simulink model "LineFollowing3kush"  (R2023a)
settings: Solver=FixedStepDiscrete  StartTime=0.0  StopTime=500  FixedStep=0.01  RelTol=1e-3
undefined symbols (not defined in the file or in its folder): InputPWM, WheelSpeed
libraries: arduinolib x10, commrandsrc3 x1, arduinosensorlib x1
settings Model: SimulationMode=external  ExtModeTrigDuration=2  Creator=Boitumelo  LastModifiedBy=ankus
settings SolverCC: AutoInsertRateTranBlk=on
settings OptimizationCC: EnhancedBackFolding=on  PassReuseOutputArgsAs=Individual arguments  ZeroExternalMemoryAtStartup=off  ZeroInternalMemoryAtStartup=off  MaxStackSize=64  OptimizeBlockOrder=speed  DifferentSizesBufferReuse=on  OptimizationCustomize=off  EfficientTunableParamExpr=on
settings DebuggingCC: ParameterTunabilityLossMsg=error  UnconnectedInputMsg=warning  UnconnectedOutputMsg=warning  UnconnectedLineMsg=warning
settings HardwareCC: ProdBitPerPointer=32  ProdBitPerSizeT=32  ProdBitPerPtrDiffT=32  ProdLargestAtomicInteger=Long  ProdLargestAtomicFloat=Double  ProdWordSize=32  ProdHWDeviceType=ARM Compatible->ARM Cortex
settings SFSimCC: MATLABDynamicMemAlloc=off
settings RTWCC: Description=Embedded Coder  SystemTargetFile=ert.tlc  HardwareBoard=Arduino Nano 33 IoT  TemplateMakefile=ert_default_tmf  GenerateReport=on  RTWVerbose=off  RTWUseSimCustomCode=on  Toolchain=Arduino ARM  BuildConfiguration=Faster Runs  DLArmComputeVersion=19.05
settings CodeAppCC: ForceParamTrailComments=on  IgnoreCustomStorageClasses=off  MaxIdLength=32  OperatorAnnotations=on  SimulinkDataObjDesc=on  SFDataObjDesc=on  InsertBlockDesc=on
settings ERTTargetCC: SupportContinuousTime=on  SupportVariableSizeSignals=on  ExtModeTransport=3  ExtModeStaticAlloc=on  ExtModeAutomaticAllocSize=off  ExtModeStaticAllocSize=8192  ExtModeMexFile=ext_xcp  ExtModeIntrfLevel=Level2 - Open

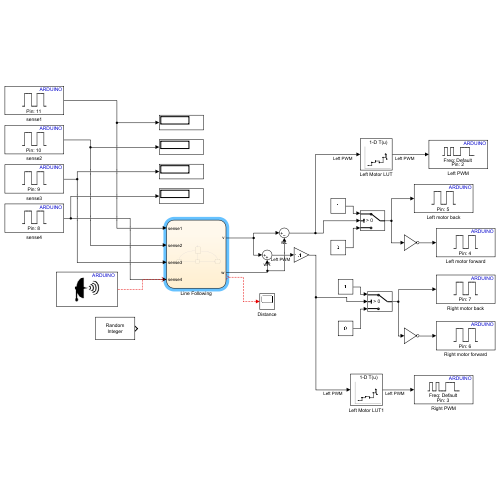
[thumbnail: Simulink's stored preview of the top-level diagram]
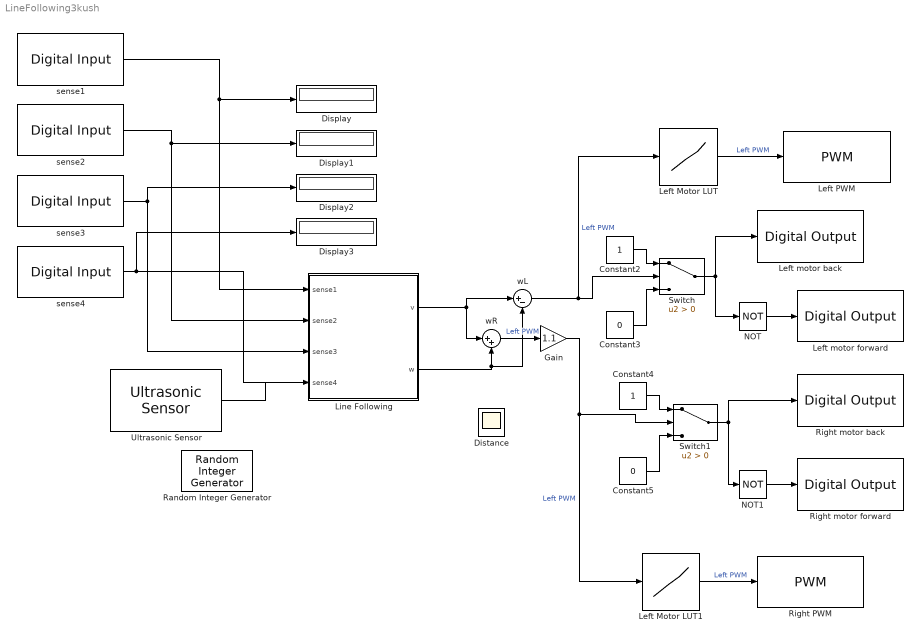
== system LineFollowing3kush ==
  Constant2 : Constant
  Constant3 : Constant  Value=0
  Constant4 : Constant
  Constant5 : Constant  Value=0
  Display{,1..3} (4 alike) : Display
  Distance : Scope
  Gain : Gain  Gain=1.1
  Left Motor LUT : Lookup_n-D  NumberOfTableDimensions=1  BreakpointsForDimension1=WheelSpeed  Table=InputPWM  InterpMethod=Nearest  ExtrapMethod=Clip  InternalRulePriority=Speed  RndMeth=Simplest
  Left Motor LUT1 : Lookup_n-D  NumberOfTableDimensions=1  BreakpointsForDimension1=WheelSpeed  Table=InputPWM  InterpMethod=Nearest  ExtrapMethod=Clip  InternalRulePriority=Speed  RndMeth=Simplest
  Left PWM : arduinolib/PWM  pinNumber=2  frequencyType=Default  desiredFrequency=490.2  achievableFrequency=490.2
  Left motor back : arduinolib/Digital Output  pinNumber=5  Direction=output  blockPlatform=arduino
  Left motor forward : arduinolib/Digital Output  pinNumber=4  Direction=output  blockPlatform=arduino
  Line Following : Stateflow chart  TreatAsAtomicUnit=on
      settings: PortSchema="{\"entries\":[{\"content\":{\"sides\":[{\"content\":{\"connectorIds\":[\"In4\",\"In2\",\"In1\",\"In3\"]},\"type\":\"ConnectorPlacement.EquallySpacedRectSide\",\"uuid\":\"3c924089-815b-40f2-b705-e6f66b84a150\"},{\"content\":{\"connectorIds\":[\"Out1\",\"Out2\"],\"side\":\"RIGHT\"},\"type\":\"ConnectorPlacement.EquallySpacedRectSide\",\"uuid\":\"d97906a3-7a34-4a96-a938-e8013b4137fd\"},{\"content\":{\"side\":\"TOP\"},\"type\":\"ConnectorPlacement.EquallySpacedRectSide\",\"uuid\":\"ab6da0b6-50e7-4a77-9ad9-89c802a4b943\"},{\"content\":{\"side\":\"BOTTOM\"},\"type\":\"ConnectorPlacement.EquallySpacedRectSide\",\"uuid\":\"37180fb4-5957-42f4-9c3a-063e4539371b\"}]},\"type\":\"ConnectorPlacement.EquallySpacedConnector\",\"uuid\":\"1e5cd3fb-bfdf-4f54-ace9-00fd0673d45b\"}],\"packageUris\":[\"http://schema.mathworks.com/mf0/Connector/R2020b\"],\"version\":\"1.0\"}"
  NOT : Logic  Operator=NOT  IconShape=distinctive  AllPortsSameDT=off  OutDataTypeStr=boolean
  NOT1 : Logic  Operator=NOT  IconShape=distinctive  AllPortsSameDT=off  OutDataTypeStr=boolean
  Random Integer Generator : commrandsrc3/Random Integer Generator  SetSize=2  SeedSource=Auto  Seed=0  SampleTime=1  SamplesPerFrame=1  OutputDataType=boolean  SimulateUsing=Interpreted execution
  Right PWM : arduinolib/PWM  pinNumber=3  frequencyType=Default  desiredFrequency=490.2  achievableFrequency=490.2
  Right motor back : arduinolib/Digital Output  pinNumber=7  Direction=output  blockPlatform=arduino
  Right motor forward : arduinolib/Digital Output  pinNumber=6  Direction=output  blockPlatform=arduino
  Switch : Switch  Criteria=u2 > Threshold  SaturateOnIntegerOverflow=off  InputSameDT=off
  Switch1 : Switch  Criteria=u2 > Threshold  SaturateOnIntegerOverflow=off  InputSameDT=off
  Ultrasonic Sensor : arduinosensorlib/Ultrasonic Sensor  NumSignalPins=2  TrigPin=13  EchoPin=12  SignalPin=3  SampleTime_=0.01  blockPlatform=ARDUINO
  sense1 : arduinolib/Digital Input  pinNumber=11  mode=Default  Direction=input  SampleTime=0.1  blockPlatform=arduino
  sense2 : arduinolib/Digital Input  pinNumber=10  mode=Default  Direction=input  SampleTime=0.1  blockPlatform=arduino
  sense3 : arduinolib/Digital Input  pinNumber=9  mode=Default  Direction=input  SampleTime=0.1  blockPlatform=arduino
  sense4 : arduinolib/Digital Input  pinNumber=8  mode=Default  Direction=input  SampleTime=0.1  blockPlatform=arduino
  wL : Sum  Inputs=|+-
  wR : Sum  Inputs=|++
  wires:
  Line Following/2(w) -> wL/2, wR/2
  Line Following/1(v) -> wL/1, wR/1
  sense1/1 -> Display/1, Line Following/4(sense1)
  sense2/1 -> Display1/1, Line Following/2(sense2)
  sense3/1 -> Display2/1, Line Following/1(sense3)
  sense4/1 -> Display3/1, Line Following/3(sense4)
  Ultrasonic Sensor/1 -> ?
  Constant3/1 -> Switch/3
  Constant2/1 -> Switch/1
  Switch/1 -> NOT/1, Left motor back/1
  NOT1/1 -> Right motor forward/1
  Gain/1 -> Switch1/2, Left Motor LUT1/1  "Left PWM"
  Switch1/1 -> NOT1/1, Right motor back/1
  Constant5/1 -> Switch1/3
  Constant4/1 -> Switch1/1
  wL/1 -> Switch/2, Left Motor LUT/1  "Left PWM"
  Left Motor LUT1/1 -> Right PWM/1  "Left PWM"
  Left Motor LUT/1 -> Left PWM/1  "Left PWM"
  NOT/1 -> Left motor forward/1
  ? -> Distance/1
  wR/1 -> Gain/1  "Left PWM"

== stateflow chart LineFollowing3kush/Line Following ==
  state Drive
    entry:
    v=2.5;
    w=0;
    i;
    n;
    data1;
    block=4;
  state WaitASec
    entry:
    v=0;
    w=0;
  state TurnRight
    entry:
    v=0;
    w=-5;
  state TurnLeft
    entry:
    v=0;
    w=5;
  (default) -> Drive
  TurnLeft -> Drive : [after(0.11,sec)&&sense3==0]
  TurnRight -> Drive : [after(0.1,sec)&&sense2==0]
  Drive -> WaitASec : [sense2~=0||sense3~=0]
  WaitASec -> TurnLeft [order 1] : [sense1==1||sense2==0&&sense4==1]
  WaitASec -> TurnRight [order 2] : [sense1==1&&sense3==0||sense4==0]
  data: v output; w output; sense3 input; sense2 input; sense4 input; sense1 input; i local =0; n local =1; data1 local =100; block local
